simulink model "dynamics"  (R2023a)
settings: Solver=ode4  StartTime=0.0  StopTime=t_duration  FixedStep=dt  MaxStep=max_step_size  RelTol=relative_tolerance
undefined symbols (not defined in the file): chief, deputy1, deputy2, dt, environment
settings Model: Creator=ndelurgio  LastModifiedBy=ndelurgio

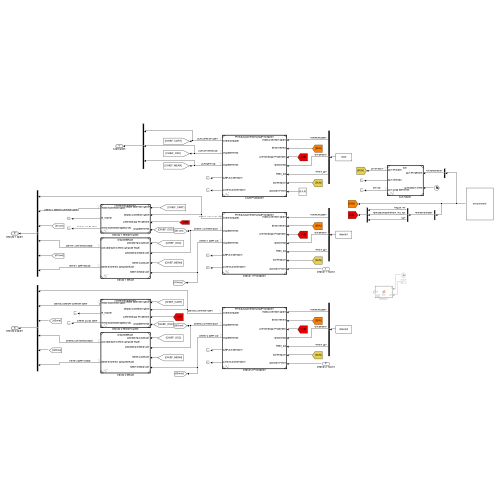
[thumbnail: Simulink's stored preview of the top-level diagram]
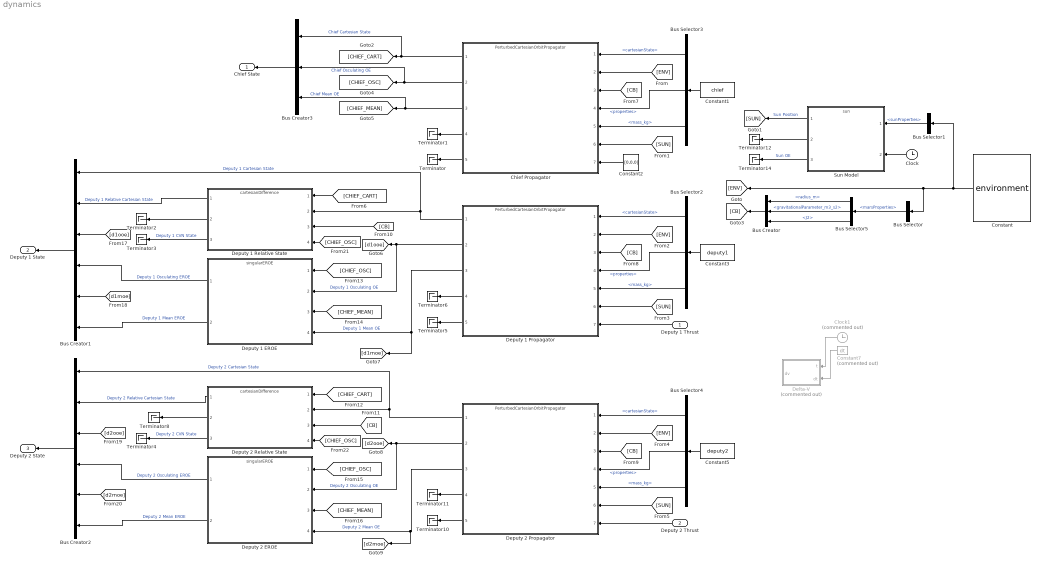
== system dynamics ==
  Deputy 1 Thrust : Inport
  Deputy 2 Thrust : Inport  Port=2
  Bus Creator : BusCreator  Inputs=3  OutDataTypeStr=Bus: planetProperties  NonVirtualBus=on
      settings: InheritFromInputs=off
  Bus Creator1 : BusCreator  Inputs=6  OutDataTypeStr=Bus: deputy1state  NonVirtualBus=on
      settings: InheritFromInputs=off
  Bus Creator2 : BusCreator  Inputs=6  OutDataTypeStr=Bus: deputy2state  NonVirtualBus=on
      settings: InheritFromInputs=off
  Bus Creator3 : BusCreator  Inputs=3  OutDataTypeStr=Bus: chiefState  NonVirtualBus=on
      settings: InheritFromInputs=off
  Bus Selector : BusSelector  OutputSignals=marsProperties
  Bus Selector1 : BusSelector  OutputSignals=sunProperties
  Bus Selector2 : BusSelector  OutputSignals=initialConditions.cartesianState,properties,initialConditions.mass_kg
  Bus Selector3 : BusSelector  OutputSignals=initialConditions.cartesianState,properties,initialConditions.mass_kg
  Bus Selector4 : BusSelector  OutputSignals=initialConditions.cartesianState,properties,initialConditions.mass_kg
  Bus Selector5 : BusSelector  OutputSignals=radius_m,gravitationalParameter_m3_s2,J2
  Chief Propagator : ModelReference  ModelNameDialog=PerturbedCartesianOrbitPropagator  SimulationMode=Normal  ModelReferenceVersion=1.197
  Clock : Clock
  Clock1 : Clock  Commented=on
  Constant : Constant  Value=environment  OutDataTypeStr=Bus: environmentBus
  Constant1 : Constant  Value=chief  OutDataTypeStr=Bus: chiefBus
  Constant2 : Constant  Value=[0,0,0]
  Constant3 : Constant  Value=deputy1  OutDataTypeStr=Bus: deputy1Bus
  Constant5 : Constant  Value=deputy2  OutDataTypeStr=Bus: deputy2Bus
  Constant7 : Constant  Commented=on  Value=dt
  Delta-V : MATLAB Function  Commented=on  TreatAsAtomicUnit=on
  Deputy 1 EROE : ModelReference  ModelNameDialog=singularEROE  SimulationMode=Normal  ModelReferenceVersion=1.18
  Deputy 1 Propagator : ModelReference  ModelNameDialog=PerturbedCartesianOrbitPropagator  SimulationMode=Normal  ModelReferenceVersion=1.197
  Deputy 1 Relative State : ModelReference  ModelNameDialog=cartesianDifference  SimulationMode=Normal  ModelReferenceVersion=1.42
  Deputy 2 EROE : ModelReference  ModelNameDialog=singularEROE  SimulationMode=Normal  ModelReferenceVersion=1.18
  Deputy 2 Propagator : ModelReference  ModelNameDialog=PerturbedCartesianOrbitPropagator  SimulationMode=Normal  ModelReferenceVersion=1.197
  Deputy 2 Relative State : ModelReference  ModelNameDialog=cartesianDifference  SimulationMode=Normal  ModelReferenceVersion=1.42
  Sun Model : ModelReference  ModelNameDialog=sun  SimulationMode=Normal  ModelReferenceVersion=1.22
  Terminator{,1..6,8,10..12,14} (12 alike) : Terminator
  Chief State : Outport  OutDataTypeStr=Bus: chiefState  BusOutputAsStruct=on
  Deputy 1 State : Outport  Port=2  OutDataTypeStr=Bus: deputy1state  BusOutputAsStruct=on
  Deputy 2 State : Outport  Port=3  OutDataTypeStr=Bus: deputy2state  BusOutputAsStruct=on
  wires:
  Constant/1 -> [ENV], Bus Selector/1, Bus Selector1/1
  [ENV] -> Chief Propagator/2
  Constant1/1 -> Bus Selector3/1
  Bus Selector1/1 -> Sun Model/1  "<sunProperties>"
  Clock/1 -> Sun Model/2
  Sun Model/1 -> [SUN]  "Sun Position"
  [SUN] -> Chief Propagator/6
  Constant2/1 -> Chief Propagator/7
  Chief Propagator/5 -> Terminator/1
  Chief Propagator/4 -> Terminator1/1
  Chief Propagator/1 -> [CHIEF_CART], Bus Creator3/1  "Chief Cartesian State"
  Chief Propagator/2 -> [CHIEF_OSC], Bus Creator3/2  "Chief Osculating OE"
  Chief Propagator/3 -> Bus Creator3/3, [CHIEF_MEAN]  "Chief Mean OE"
  Bus Selector3/2 -> Chief Propagator/4  "<properties>"
  Bus Selector3/1 -> Chief Propagator/1  "<cartesianState>"
  Bus Selector3/3 -> Chief Propagator/5  "<mass_kg>"
  Deputy 1 Propagator/5 -> Terminator5/1
  Deputy 1 Propagator/2 -> Deputy 1 EROE/2, [d1ooe]  "Deputy 1 Osculating OE"
  Deputy 1 Propagator/1 -> Bus Creator1/1, Deputy 1 Relative State/2  "Deputy 1 Cartesian State"
  Deputy 1 Propagator/4 -> Terminator6/1
  Deputy 1 Propagator/3 -> [d1moe], Deputy 1 EROE/4  "Deputy 1 Mean OE"
  Deputy 2 Propagator/5 -> Terminator10/1
  Constant5/1 -> Bus Selector4/1
  Deputy 2 Propagator/4 -> Terminator11/1
  [CHIEF_CART] -> Deputy 1 Relative State/1
  Bus Selector/1 -> Bus Selector5/1  "<marsProperties>"
  [CB] -> Chief Propagator/3
  [ENV] -> Deputy 1 Propagator/2
  [CB] -> Deputy 1 Propagator/3
  Bus Selector2/1 -> Deputy 1 Propagator/1  "<cartesianState>"
  Bus Selector2/2 -> Deputy 1 Propagator/4  "<properties>"
  Bus Selector2/3 -> Deputy 1 Propagator/5  "<mass_kg>"
  [SUN] -> Deputy 1 Propagator/6
  Constant3/1 -> Bus Selector2/1
  [CB] -> Deputy 2 Propagator/3
  [SUN] -> Deputy 2 Propagator/6
  Bus Selector4/1 -> Deputy 2 Propagator/1  "<cartesianState>"
  [ENV] -> Deputy 2 Propagator/2
  Bus Selector4/3 -> Deputy 2 Propagator/5  "<mass_kg>"
  Deputy 2 Thrust/1 -> Deputy 2 Propagator/7
  Bus Selector4/2 -> Deputy 2 Propagator/4  "<properties>"
  [CB] -> Deputy 1 Relative State/3
  [CHIEF_CART] -> Deputy 2 Relative State/1
  [CB] -> Deputy 2 Relative State/3
  Deputy 2 Propagator/1 -> Bus Creator2/1, Deputy 2 Relative State/2  "Deputy 2 Cartesian State"
  Deputy 2 Relative State/2 -> Terminator8/1
  Deputy 1 Relative State/1 -> Bus Creator1/2  "Deputy 1 Relative Cartesian State"
  Deputy 2 Relative State/1 -> Bus Creator2/2  "Deputy 2 Relative Cartesian State"
  [CHIEF_OSC] -> Deputy 1 EROE/1
  [CHIEF_MEAN] -> Deputy 1 EROE/3
  Deputy 1 EROE/1 -> Bus Creator1/4  "Deputy 1 Osculating EROE"
  Deputy 1 EROE/2 -> Bus Creator1/6  "Deputy 1 Mean EROE"
  [CHIEF_MEAN] -> Deputy 2 EROE/3
  [CHIEF_OSC] -> Deputy 2 EROE/1
  Deputy 2 EROE/2 -> Bus Creator2/6  "Deputy 2 Mean EROE"
  Deputy 2 Propagator/3 -> [d2moe], Deputy 2 EROE/4  "Deputy 2 Mean OE"
  Deputy 2 EROE/1 -> Bus Creator2/4  "Deputy 2 Osculating EROE"
  Deputy 2 Propagator/2 -> [d2ooe], Deputy 2 EROE/2  "Deputy 2 Osculating OE"
  Bus Creator/1 -> [CB]
  Bus Selector5/1 -> Bus Creator/1  "<radius_m>"
  Bus Selector5/2 -> Bus Creator/2  "<gravitationalParameter_m3_s2>"
  Bus Selector5/3 -> Bus Creator/3  "<J2>"
  Sun Model/2 -> Terminator12/1
  Sun Model/3 -> Terminator14/1  "Sun OE"
  Deputy 1 Thrust/1 -> Deputy 1 Propagator/7
  Clock1/1 -> Delta-V/1(t)
  Constant7/1 -> Delta-V/2(dt)
  [d1ooe] -> Bus Creator1/3
  [d1moe] -> Bus Creator1/5
  Deputy 1 Relative State/2 -> Terminator2/1
  Bus Creator1/1 -> Deputy 1 State/1
  [d2ooe] -> Bus Creator2/3
  [d2moe] -> Bus Creator2/5
  Bus Creator2/1 -> Deputy 2 State/1
  Bus Creator3/1 -> Chief State/1
  [CHIEF_OSC] -> Deputy 1 Relative State/4
  [CHIEF_OSC] -> Deputy 2 Relative State/4
  Deputy 1 Relative State/3 -> Terminator3/1  "Deputy 1 CVN State"
  Deputy 2 Relative State/3 -> Terminator4/1  "Deputy 2 CVN State"

== matlab function dynamics/Delta-V ==
  data: t input; dv output; dt input
function dv = fcn(t, dt)

if abs(t-5000) <= dt
    dv = [1;0;0];
else
    dv = [0;0;0];
end

end
